simulink library "lib_fuel_converter3"  (Simulink 4.1.1)
values from neighbouring files (symbols this model uses):
  logFlag = 1    [advSACompMaskInit.m]    (also in advSACompMaskInitR13.m)
undefined symbols (not defined in the file or in its folder): air_cp, amb_tmp, cyc_mph, ex_gas_cp, fc_acc_mass, fc_base_mass, fc_c2i_th_cond, fc_c_init_tmp, fc_cl2h_eff, fc_CO2_to_FUELgps, fc_cold, fc_cold_tmp, fc_cp, fc_ct_trq, fc_emisv, fc_ext_sarea, fc_fuel_den, fc_fuel_lhv, fc_h2x_th_cond, fc_h_air_flow, fc_h_cp, fc_h_init_tmp, fc_hood_emisv, fc_hood_sarea, fc_i2x_th_cond, fc_i_init_tmp, fc_inertia, fc_map_spd, fc_map_trq, fc_max_trq, fc_nn_model_name, fc_pwr_scale, fc_spd_scale, fc_trq_scale, fc_tstat, fc_x_init_tmp, fd_ratio, gb_num_init, gb_ratio, generalName, pow, vc_idle_bool, vc_idle_spd, vc_key_on, veh_glider_mass, wh_radius
libraries: lib_fuel_converter3 x4, lib_etc x4, lib_fuel_converter x2, lib_fuel_converter2 x1
(part 1 of 9)
settings Model: LastModifiedBy=mokeefe

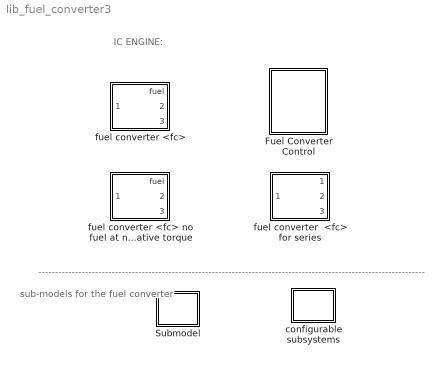
== system lib_fuel_converter3 ==
  note: --------------------------------------------------------------------------------------------------------------------
  note: sub-models
      | for the fuel converter
  note: IC ENGINE:
  Fuel Converter Control : Subsystem
      settings: RTWFcnNameOpts=Auto  RTWFileNameOpts=Auto
  Submodel : Subsystem
      settings: RTWFcnNameOpts=Auto  RTWFileNameOpts=Auto
  configurable subsystems : Subsystem
      settings: RTWFcnNameOpts=Auto  RTWFileNameOpts=Auto
  fuel converter  <fc> for series : Subsystem  mask(Stand-Alone IC ENGINE Mask (Series Hybrid)){generalName='fc', logPick=Log, initFileName={}, modCell={}, imgFileName='bdi_fc.jpg', DEBUG=OFF}
      mask prompts: generalName "General Name of this Component [char]"; logPick "Log Variables to Workspace?"; initFileName "Initialization File(s) [cell array of char]"; modCell "Modification Cell [2 column cell array of param and val]"; imgFileName "Icon image file name [char--evaluated]"
      mask init:
      | % initialization via m-file script
      | advSACompMaskInit;
      settings: RTWFcnNameOpts=Auto  RTWFileNameOpts=Auto
      mask StyleString: edit,popup(Don't Log|Log),edit,edit,edit,popup(ON|OFF)
      mask Display: image(imread(imgFileName))
  fuel converter <fc> : Subsystem  mask(Stand-Alone IC ENGINE Mask){generalName='fc', logPick=Log, initFileName={}, modCell={}, imgFileName='bdi_fc.jpg', DEBUG=OFF}
      mask prompts: generalName "General Name of this Component [char]"; logPick "Log Variables to Workspace?"; initFileName "Initialization File(s) [cell array of char]"; modCell "Modification Cell [2 column cell array of param and val]"; imgFileName "Icon image file name [char--evaluated]"
      mask init:
      | % initialization via m-file script
      | advSACompMaskInit;
      settings: RTWFcnNameOpts=Auto  RTWFileNameOpts=Auto
      mask StyleString: edit,popup(Don't Log|Log),edit,edit,edit,popup(ON|OFF)
      mask Display: image(imread(imgFileName))
  fuel converter <fc> no fuel at negative torque : Subsystem  mask(Stand-Alone IC ENGINE Mask){generalName='fc', logPick=Log, initFileName={}, modCell={}, imgFileName='bdi_fc.jpg', DEBUG=OFF}
      mask prompts: generalName "General Name of this Component [char]"; logPick "Log Variables to Workspace?"; initFileName "Initialization File(s) [cell array of char]"; modCell "Modification Cell [2 column cell array of param and val]"; imgFileName "Icon image file name [char--evaluated]"
      mask init:
      | % initialization via m-file script
      | advSACompMaskInit;
      settings: RTWFcnNameOpts=Auto  RTWFileNameOpts=Auto
      mask StyleString: edit,popup(Don't Log|Log),edit,edit,edit,popup(ON|OFF)
      mask Display: image(imread(imgFileName))

== system lib_fuel_converter3/Fuel Converter Control ==
  Fuel Converter Control conventional ic engine : Subsystem
      settings: RTWFcnNameOpts=Auto  RTWFileNameOpts=Auto

== system lib_fuel_converter3/Submodel ==
  engine inertia as a function of total vehicle inertia (generous approximation) : Subsystem  Orientation=down
      settings: RTWFcnNameOpts=Auto  RTWFileNameOpts=Auto
  veh mass calc : Subsystem
      settings: RTWFcnNameOpts=Auto  RTWFileNameOpts=Auto

== system lib_fuel_converter3/configurable subsystems ==
  fuel use and EO emis : Subsystem
      settings: RTWFcnNameOpts=Auto  RTWFileNameOpts=Auto
  fuel use and EO emis Configurable Subsystem : Subsystem  BlockChoice=fuel use and EO emis
      settings: TemplateBlock=self  MemberBlocks=fuel use and EO emis,fuel use and EO emis Neural Network Model  RTWFcnNameOpts=Auto  RTWFileNameOpts=Auto
  fuel use and EO emis Neural Network Model : Subsystem  mask{modelName=fc_nn_model_name}
      mask prompts: modelName "model no. (see help for specs)"
      mask help: Neural Network Model for Engine Fuel and Emissions Prediction
      mask init:
      | if strcmp(modelName,'1999CumminsISM370')
      |      modelNum=0;
      |      disp('Neural Net Model: 1999CumminsISM370')
      | elseif strcmp(modelName,'1994NavistarT444E')
      |      modelNum=1;
      |      disp('Neural Net Model: 1994NavistarT444E')
      | else
      |      modelNum=-1;
      |      disp('Neural Net Model: Invalid Setting!')
      |      disp('check value of fc_nn_model_name')
      | end
      settings: RTWFcnNameOpts=Auto  RTWFileNameOpts=Auto
      mask Help:
      | <h1>Neural Network Emissions Block Help</h1>
      | <h2>Introduction</h2>
      | <p>The neural network model takes engine shaft speed and torque and their time derivatives at 5 seconds and 10 seconds and predicts CO, CO2, and NOx emissions in g/s. Inputs to the model are speed (rpm) and torque (Nm). Outputs are CO, CO2, and NOx emissions in g/s.</p>
      | 
      | <p>There are neural network models trained for two engines thus far:</p>
      | <ol>
      | <li>1999 Cummins ISM 370</li>
      | <li>1994 Navistar T 444E</li>
      | </ol>
      | <p>In order to access the neural net models, one must type a string into the mask input screen. That string corresponds to:</p>
      | 
      | <table border=1>
      | <tr><td>Name</td><td>Engine</td></tr>
      | <tr><td>'1999CumminsISM370'</td><td>Cummins ISM 370</td></tr>
      | <tr><td>'1994NavistarT444E'</td><td>Navistar T 444E</td></tr>
      | </table>

== system lib_fuel_converter3/fuel converter  <fc> for series ==
  note: Internal Combustion Engine
      | for Series Powertrain
  torque and speed  req'd at engine  output shaft (Nm) : Inport  Port=1  LatchInput=off
  Model & Interface : Subsystem
      settings: RTWFcnNameOpts=Auto  RTWFileNameOpts=Auto
  fuel use : Outport  Port=1  InitialOutput=0
  EO emis info : Outport  Port=2  InitialOutput=0
  "torque and speed  avail. to driveline (Nm), (rad/s)" : Outport  Port=3  InitialOutput=0
  tag scope: fcReqOut=global, fcSensors=global
  wires:
  Model & Interface/2(fuel use) -> fuel use/1
  torque and speed  req'd at engine  output shaft (Nm)/1 -> Model & Interface/1(torque and speed  req'd at engine  output shaft (Nm))
  Model & Interface/3(EO emis info) -> EO emis info/1
  Model & Interface/4("torque and speed  avail. to driveline (Nm), (rad/s)") -> "torque and speed  avail. to driveline (Nm), (rad/s)"/1
  [fcControl] -> Model & Interface/2(control)
  Model & Interface/1(req'd out) -> [fcReqOut]
  Model & Interface/5(sensors) -> [fcSensors]

== system lib_fuel_converter3/fuel converter <fc> ==
  note: Internal Combustion Engine
  trq and spd out requested : Inport  Port=1  LatchInput=off
  Block NOTES : Subsystem
      settings: RTWFcnNameOpts=Auto  RTWFileNameOpts=Auto
      mask Display: disp('Block\nNOTES')
  IC Engine Model  &  Interface : Subsystem
      settings: RTWFcnNameOpts=Auto  RTWFileNameOpts=Auto
  help : Subsystem
      settings: OpenFcn=web(['file:\\\' which('fuel_converter.htm')]);  RTWFcnNameOpts=Auto  RTWFileNameOpts=Auto
      mask Display: image(imread('doc_man.jpg'))
  fuel : Outport  Port=1
  engine out emissions : Outport  Port=2
  trq and spd out achieved : Outport  Port=3
  tag scope: fcReqOut=global, fcSensors=global
  wires:
  trq and spd out requested/1 -> IC Engine Model  &  Interface/1(trq and spd out requested)
  [fcControl] -> IC Engine Model  &  Interface/2(control)
  IC Engine Model  &  Interface/5(sensors) -> [fcSensors]
  IC Engine Model  &  Interface/4(trq and spd out achieved) -> trq and spd out achieved/1
  IC Engine Model  &  Interface/3(engine out emissions) -> engine out emissions/1
  IC Engine Model  &  Interface/2(fuel) -> fuel/1
  IC Engine Model  &  Interface/1(req out) -> [fcReqOut]

== system lib_fuel_converter3/fuel converter <fc> no fuel at negative torque ==
  note: Internal Combustion Engine
  trq and spd out requested : Inport  Port=1  LatchInput=off
  Block NOTES : Subsystem
      settings: RTWFcnNameOpts=Auto  RTWFileNameOpts=Auto
      mask Display: disp('Block\nNOTES')
  IC Engine Model  &  Interface : Subsystem
      settings: RTWFcnNameOpts=Auto  RTWFileNameOpts=Auto
  help : Subsystem
      settings: OpenFcn=web(['file:\\\' which('fuel_converter.htm')]);  RTWFcnNameOpts=Auto  RTWFileNameOpts=Auto
      mask Display: image(imread('doc_man.jpg'))
  fuel : Outport  Port=1
  engine out emissions : Outport  Port=2
  trq and spd out achieved : Outport  Port=3
  tag scope: fcReqOut=global, fcSensors=global
  wires:
  trq and spd out requested/1 -> IC Engine Model  &  Interface/1(trq and spd out requested)
  [fcControl] -> IC Engine Model  &  Interface/2(control)
  IC Engine Model  &  Interface/5(sensors) -> [fcSensors]
  IC Engine Model  &  Interface/4(trq and spd out achieved) -> trq and spd out achieved/1
  IC Engine Model  &  Interface/3(engine out emissions) -> engine out emissions/1
  IC Engine Model  &  Interface/2(fuel) -> fuel/1
  IC Engine Model  &  Interface/1(req out) -> [fcReqOut]

== system lib_fuel_converter3/Fuel Converter Control/Fuel Converter Control conventional ic engine ==
  conventional IC engine : Subsystem
      settings: RTWFcnNameOpts=Auto  RTWFileNameOpts=Auto

== system lib_fuel_converter3/Submodel/engine inertia as a function of total vehicle inertia (generous approximation) ==
  Product : Product  Orientation=down  Inputs=*/  Multiplication=Element-wise(.*)  SaturateOnIntegerOverflow=on
  Sum : Sum  Orientation=down  Inputs=++|  SaturateOnIntegerOverflow=on
  engine inertia as a fraction of total vehicle inertia  (generous approximation)--denomenator : Fcn  Orientation=down  Expr=fc_inertia*(u*fd_ratio/wh_radius)^2
  engine inertia as a fraction of total vehicle inertia  (generous approximation)--numerator : Fcn  Orientation=down  Expr=fc_inertia*(u*fd_ratio/wh_radius)^2
  veh mass calc : lib_fuel_converter3/Submodel/veh mass calc
      settings: RTWFcnNameOpts=Auto  RTWFileNameOpts=Auto
  Out1 : Outport  Orientation=down  Port=1
  wires:
  Product/1 -> Out1/1
  Sum/1 -> Product/2
  engine inertia as a fraction of total vehicle inertia  (generous approximation)--numerator/1 -> Product/1
  engine inertia as a fraction of total vehicle inertia  (generous approximation)--denomenator/1 -> Sum/2
  veh mass calc/1 -> Sum/1
  [gear_ratio] -> engine inertia as a fraction of total vehicle inertia  (generous approximation)--denomenator/1, engine inertia as a fraction of total vehicle inertia  (generous approximation)--numerator/1

== system lib_fuel_converter3/Submodel/veh mass calc ==
  Out1 : Outport  Port=1
  wires:
  [current_veh_mass] -> Out1/1

== system lib_fuel_converter3/configurable subsystems/fuel use and EO emis ==
  T (Nm) : Inport  Port=1  LatchInput=off
  w (rad/s) : Inport  Port=2  LatchInput=off
  (gal/s) : Gain  Gain=1/fc_fuel_den*61.02/231  Multiplication=Element-wise(K.*u)  SaturateOnIntegerOverflow=on
  Block NOTES : Subsystem
      settings: RTWFcnNameOpts=Auto  RTWFileNameOpts=Auto
      mask Display: disp('Block\nNOTES')
  Demux : Demux  Outputs=2  BusSelectionMode=off
  HOT engine maps : Subsystem  TreatAsAtomicUnit=on
      settings: RTWFcnNameOpts=Auto  RTWFileNameOpts=Auto
  Integrator : Integrator  ExternalReset=none  InitialConditionSource=internal  InitialCondition=0  LimitOutput=off  UpperSaturationLimit=inf  LowerSaturationLimit=-inf  ShowSaturationPort=off  ShowStatePort=off  AbsoluteTolerance=auto
  Mux4 : Mux  Inputs=[1 4 1 1 1]
      settings: DisplayOption=none
  Mux5 : Mux  Inputs=[1 4 ]
      settings: DisplayOption=none
  Selector3 : Selector  Orientation=down  InputType=Vector  ElementSrc=Internal  Elements=2  RowSrc=Internal  Rows=1  ColumnSrc=Internal  Columns=1  InputPortWidth=4
  Terminator : Terminator
  enhancedToWorkspace1 : Subsystem  mask(enhancedToWorkspace){generalName=generalName, specificName=th_pwr, logFlag=logFlag}
      mask prompts: generalName "General Name [char-evaluated]"; specificName "Specific Name [char-literal]"; logFlag "Enable flag (1=on,0=off)"
      mask help: A wrapper for the Simulink "To Workspace" block that allows you to evaluate the name of the variable to log to workspace. This is useful to avoid the double logging errors that occur when you pull in two library models that attempt to log to the same variable.
      mask init:
      | enhancedToWsMaker
      settings: CopyFcn=breakLinkCopyFcn  RTWFcnNameOpts=Auto  RTWFileNameOpts=Auto
      mask Display: disp([generalName,'_',specificName])
  enhancedToWorkspace10 : Subsystem  mask(enhancedToWorkspace){generalName=generalName, specificName=ex_gas_tmp, logFlag=logFlag}
      mask prompts: generalName "General Name [char-evaluated]"; specificName "Specific Name [char-literal]"; logFlag "Enable flag (1=on,0=off)"
      mask help: A wrapper for the Simulink "To Workspace" block that allows you to evaluate the name of the variable to log to workspace. This is useful to avoid the double logging errors that occur when you pull in two library models that attempt to log to the same variable.
      mask init:
      | enhancedToWsMaker
      settings: CopyFcn=breakLinkCopyFcn  RTWFcnNameOpts=Auto  RTWFileNameOpts=Auto
      mask Display: disp([generalName,'_',specificName])
  enhancedToWorkspace11 : Subsystem  mask(enhancedToWorkspace){generalName=generalName, specificName=ex_th_pwr, logFlag=logFlag}
      mask prompts: generalName "General Name [char-evaluated]"; specificName "Specific Name [char-literal]"; logFlag "Enable flag (1=on,0=off)"
      mask help: A wrapper for the Simulink "To Workspace" block that allows you to evaluate the name of the variable to log to workspace. This is useful to avoid the double logging errors that occur when you pull in two library models that attempt to log to the same variable.
      mask init:
      | enhancedToWsMaker
      settings: CopyFcn=breakLinkCopyFcn  RTWFcnNameOpts=Auto  RTWFileNameOpts=Auto
      mask Display: disp([generalName,'_',specificName])
  enhancedToWorkspace12 : Subsystem  Orientation=left  mask(enhancedToWorkspace){generalName=generalName, specificName=clt_tmp, logFlag=logFlag}
      mask prompts: generalName "General Name [char-evaluated]"; specificName "Specific Name [char-literal]"; logFlag "Enable flag (1=on,0=off)"
      mask help: A wrapper for the Simulink "To Workspace" block that allows you to evaluate the name of the variable to log to workspace. This is useful to avoid the double logging errors that occur when you pull in two library models that attempt to log to the same variable.
      mask init:
      | enhancedToWsMaker
      settings: CopyFcn=breakLinkCopyFcn  RTWFcnNameOpts=Auto  RTWFileNameOpts=Auto
      mask Display: disp([generalName,'_',specificName])
  enhancedToWorkspace2 : Subsystem  mask(enhancedToWorkspace){generalName=generalName, specificName=o2_flow, logFlag=logFlag}
      mask prompts: generalName "General Name [char-evaluated]"; specificName "Specific Name [char-literal]"; logFlag "Enable flag (1=on,0=off)"
      mask help: A wrapper for the Simulink "To Workspace" block that allows you to evaluate the name of the variable to log to workspace. This is useful to avoid the double logging errors that occur when you pull in two library models that attempt to log to the same variable.
      mask init:
      | enhancedToWsMaker
      settings: CopyFcn=breakLinkCopyFcn  RTWFcnNameOpts=Auto  RTWFileNameOpts=Auto
      mask Display: disp([generalName,'_',specificName])
  enhancedToWorkspace3 : Subsystem  mask(enhancedToWorkspace){generalName=generalName, specificName=r_th_pwr, logFlag=logFlag}
      mask prompts: generalName "General Name [char-evaluated]"; specificName "Specific Name [char-literal]"; logFlag "Enable flag (1=on,0=off)"
      mask help: A wrapper for the Simulink "To Workspace" block that allows you to evaluate the name of the variable to log to workspace. This is useful to avoid the double logging errors that occur when you pull in two library models that attempt to log to the same variable.
      mask init:
      | enhancedToWsMaker
      settings: CopyFcn=breakLinkCopyFcn  RTWFcnNameOpts=Auto  RTWFileNameOpts=Auto
      mask Display: disp([generalName,'_',specificName])
  enhancedToWorkspace5 : Subsystem  mask(enhancedToWorkspace){generalName=generalName, specificName=h_th_pwr, logFlag=logFlag}
      mask prompts: generalName "General Name [char-evaluated]"; specificName "Specific Name [char-literal]"; logFlag "Enable flag (1=on,0=off)"
      mask help: A wrapper for the Simulink "To Workspace" block that allows you to evaluate the name of the variable to log to workspace. This is useful to avoid the double logging errors that occur when you pull in two library models that attempt to log to the same variable.
      mask init:
      | enhancedToWsMaker
      settings: CopyFcn=breakLinkCopyFcn  RTWFcnNameOpts=Auto  RTWFileNameOpts=Auto
      mask Display: disp([generalName,'_',specificName])
  enhancedToWorkspace6 : Subsystem  mask(enhancedToWorkspace){generalName=generalName, specificName=tmp, logFlag=logFlag}
      mask prompts: generalName "General Name [char-evaluated]"; specificName "Specific Name [char-literal]"; logFlag "Enable flag (1=on,0=off)"
      mask help: A wrapper for the Simulink "To Workspace" block that allows you to evaluate the name of the variable to log to workspace. This is useful to avoid the double logging errors that occur when you pull in two library models that attempt to log to the same variable.
      mask init:
      | enhancedToWsMaker
      settings: CopyFcn=breakLinkCopyFcn  RTWFcnNameOpts=Auto  RTWFileNameOpts=Auto
      mask Display: disp([generalName,'_',specificName])
  enhancedToWorkspace7 : Subsystem  mask(enhancedToWorkspace){generalName=generalName, specificName=fuel_rate, logFlag=logFlag}
      mask prompts: generalName "General Name [char-evaluated]"; specificName "Specific Name [char-literal]"; logFlag "Enable flag (1=on,0=off)"
      mask help: A wrapper for the Simulink "To Workspace" block that allows you to evaluate the name of the variable to log to workspace. This is useful to avoid the double logging errors that occur when you pull in two library models that attempt to log to the same variable.
      mask init:
      | enhancedToWsMaker
      settings: CopyFcn=breakLinkCopyFcn  RTWFcnNameOpts=Auto  RTWFileNameOpts=Auto
      mask Display: disp([generalName,'_',specificName])
  enhancedToWorkspace8 : Subsystem  mask(enhancedToWorkspace){generalName=generalName, specificName=emis_eo, logFlag=logFlag}
      mask prompts: generalName "General Name [char-evaluated]"; specificName "Specific Name [char-literal]"; logFlag "Enable flag (1=on,0=off)"
      mask help: A wrapper for the Simulink "To Workspace" block that allows you to evaluate the name of the variable to log to workspace. This is useful to avoid the double logging errors that occur when you pull in two library models that attempt to log to the same variable.
      mask init:
      | enhancedToWsMaker
      settings: CopyFcn=breakLinkCopyFcn  RTWFcnNameOpts=Auto  RTWFileNameOpts=Auto
      mask Display: disp([generalName,'_',specificName])
  enhancedToWorkspace9 : Subsystem  mask(enhancedToWorkspace){generalName=generalName, specificName=ex_gas_flow, logFlag=logFlag}
      mask prompts: generalName "General Name [char-evaluated]"; specificName "Specific Name [char-literal]"; logFlag "Enable flag (1=on,0=off)"
      mask help: A wrapper for the Simulink "To Workspace" block that allows you to evaluate the name of the variable to log to workspace. This is useful to avoid the double logging errors that occur when you pull in two library models that attempt to log to the same variable.
      mask init:
      | enhancedToWsMaker
      settings: CopyFcn=breakLinkCopyFcn  RTWFcnNameOpts=Auto  RTWFileNameOpts=Auto
      mask Display: disp([generalName,'_',specificName])
  fc temp : Subsystem
      settings: RTWFcnNameOpts=Auto  RTWFileNameOpts=Auto
  fc temp correct : Subsystem  TreatAsAtomicUnit=on
      settings: RTWFcnNameOpts=Auto  RTWFileNameOpts=Auto
  cumulative fuel  use (gal) : Outport  Port=1  InitialOutput=0
  "FC ON?, EOem, MFex, Tex, O2ex" : Outport  Port=2  InitialOutput=0
  Vv,Tfc : Outport  Port=3  InitialOutput=0
  tag scope: fc_clt_tmp=scoped
  wires:
  [key_on] -> fc temp/2(key ON?)
  [engine_on] -> fc temp/3(fc ON?), fc temp correct/Enable, Mux4/1, HOT engine maps/Enable
  fc temp correct/2(EO emis (g/s)) -> Mux4/2, enhancedToWorkspace8/1(In1)
  Demux/2 -> enhancedToWorkspace5/1(In1)
  Demux/1 -> enhancedToWorkspace3/1(In1)
  fc temp/2(Qfc r,h) -> Demux/1
  HOT engine maps/1(fc heat (W)) -> fc temp/4(Qfc (W)), enhancedToWorkspace1/1(In1)
  Selector3/1 -> fc temp correct/1(Coolant T (C)), [fc_clt_tmp], enhancedToWorkspace12/1(In1)
  HOT engine maps/7(ex heat (W)) -> enhancedToWorkspace11/1(In1)
  fc temp/1(Tfc_old  (C)) -> Terminator/1
  fc temp/3(Tfc  (C)) -> Mux5/2, enhancedToWorkspace6/1(In1), Selector3/1
  HOT engine maps/3(HOT emis (g/s)) -> fc temp correct/3(HOT emis (g/s))
  HOT engine maps/2(HOT fuel use (g/s)) -> fc temp correct/2(HOT fuel use (g/s))
  (gal/s)/1 -> Integrator/1
  Integrator/1 -> cumulative fuel  use (gal)/1
  HOT engine maps/5(Ex Gas Temp (C)) -> Mux4/4, enhancedToWorkspace10/1(In1)
  HOT engine maps/4(Ex Gas Flow (g/s)) -> Mux4/3, enhancedToWorkspace9/1(In1)
  [v_prev] -> fc temp/1(veh spd (m/s)), Mux5/1
  Mux5/1 -> Vv,Tfc/1
  Mux4/1 -> "FC ON?, EOem, MFex, Tex, O2ex"/1
  w (rad/s)/1 -> fc temp correct/5(w (rad/s)), HOT engine maps/2(w (rad/s))
  T (Nm)/1 -> fc temp correct/4(T (Nm)), HOT engine maps/1(T (Nm))
  HOT engine maps/6(O2 exhaust (g/s)) -> Mux4/5, enhancedToWorkspace2/1(In1)
  fc temp correct/1(fuel use (g/s)) -> (gal/s)/1, enhancedToWorkspace7/1(In1)

== system lib_fuel_converter3/configurable subsystems/fuel use and EO emis Configurable Subsystem ==
  T (Nm) : Inport  Port=1  LatchInput=off
  w (rad/s) : Inport  Port=2  LatchInput=off
  fuel use and EO emis : lib_fuel_converter3/configurable subsystems/fuel use and EO emis
      settings: RTWFcnNameOpts=Auto  RTWFileNameOpts=Auto
  cumulative fuel  use (gal) : Outport  Port=1
  "FC ON?, EOem, MFex, Tex, O2ex" : Outport  Port=2
  Vv,Tfc : Outport  Port=3
  wires:
  T (Nm)/1 -> fuel use and EO emis/1
  w (rad/s)/1 -> fuel use and EO emis/2
  fuel use and EO emis/1 -> cumulative fuel  use (gal)/1
  fuel use and EO emis/2 -> "FC ON?, EOem, MFex, Tex, O2ex"/1
  fuel use and EO emis/3 -> Vv,Tfc/1

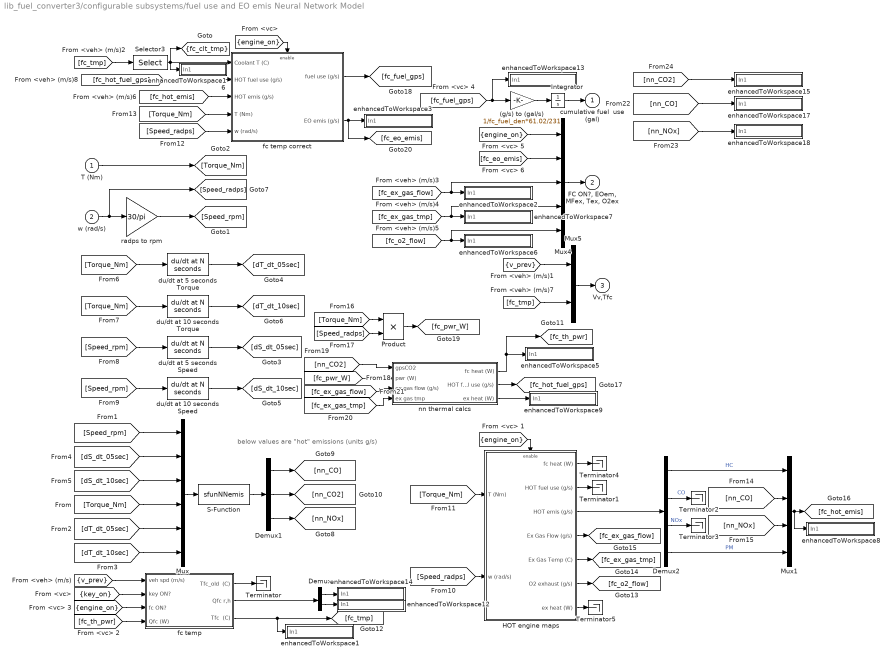
== system lib_fuel_converter3/configurable subsystems/fuel use and EO emis Neural Network Model ==
  note: below values are "hot" emissions
      | (units g/s)
  T (Nm) : Inport  Port=1  LatchInput=off
  w (rad/s) : Inport  Port=2  LatchInput=off
  (g/s) to (gal/s) : Gain  Gain=1/fc_fuel_den*61.02/231  Multiplication=Element-wise(K.*u)  SaturateOnIntegerOverflow=on
  Demux : Demux  Outputs=2  BusSelectionMode=off
  Demux1 : Demux  Outputs=3  BusSelectionMode=off
  Demux2 : Demux  Outputs=4  BusSelectionMode=off
  HOT engine maps : Subsystem  TreatAsAtomicUnit=on
      settings: RTWFcnNameOpts=Auto  RTWFileNameOpts=Auto
  Integrator : Integrator  ExternalReset=none  InitialConditionSource=internal  InitialCondition=0  LimitOutput=off  UpperSaturationLimit=inf  LowerSaturationLimit=-inf  ShowSaturationPort=off  ShowStatePort=off  AbsoluteTolerance=auto
  Mux : Mux  Inputs=6
  Mux1 : Mux  Inputs=4
  Mux4 : Mux  Inputs=[1 4 1 1 1]
      settings: DisplayOption=none
  Mux5 : Mux  Inputs=[1 4 ]
      settings: DisplayOption=none
  Product : Product  Inputs=2  Multiplication=Element-wise(.*)  SaturateOnIntegerOverflow=on
  S-Function : S-Function  FunctionName=sfunNNemis  Parameters=modelNum  PortCounts=[]  SFunctionModules=''
  Selector3 : Selector  InputType=Vector  ElementSrc=Internal  Elements=2  RowSrc=Internal  Rows=1  ColumnSrc=Internal  Columns=1  InputPortWidth=4
  Terminator{,1..5} (6 alike) : Terminator
  du/dt at 10 seconds Speed : lib_etc/du//dt at N seconds  delay=10
  du/dt at 10 seconds Torque : lib_etc/du//dt at N seconds  delay=10
  du/dt at 5 seconds Speed : lib_etc/du//dt at N seconds  delay=5
  du/dt at 5 seconds Torque : lib_etc/du//dt at N seconds  delay=5
  enhancedToWorkspace1 : Subsystem  mask(enhancedToWorkspace){generalName=generalName, specificName=tmp, logFlag=logFlag}
      mask prompts: generalName "General Name [char-evaluated]"; specificName "Specific Name [char-literal]"; logFlag "Enable flag (1=on,0=off)"
      mask help: A wrapper for the Simulink "To Workspace" block that allows you to evaluate the name of the variable to log to workspace. This is useful to avoid the double logging errors that occur when you pull in two library models that attempt to log to the same variable.
      mask init:
      | enhancedToWsMaker
      settings: CopyFcn=breakLinkCopyFcn  RTWFcnNameOpts=Auto  RTWFileNameOpts=Auto
      mask Display: disp([generalName,'_',specificName])
  enhancedToWorkspace12 : Subsystem  mask(enhancedToWorkspace){generalName=generalName, specificName=h_th_pwr, logFlag=logFlag}
      mask prompts: generalName "General Name [char-evaluated]"; specificName "Specific Name [char-literal]"; logFlag "Enable flag (1=on,0=off)"
      mask help: A wrapper for the Simulink "To Workspace" block that allows you to evaluate the name of the variable to log to workspace. This is useful to avoid the double logging errors that occur when you pull in two library models that attempt to log to the same variable.
      mask init:
      | enhancedToWsMaker
      settings: CopyFcn=breakLinkCopyFcn  RTWFcnNameOpts=Auto  RTWFileNameOpts=Auto
      mask Display: disp([generalName,'_',specificName])
  enhancedToWorkspace13 : Subsystem  mask(enhancedToWorkspace){generalName=generalName, specificName=fuel_rate, logFlag=logFlag}
      mask prompts: generalName "General Name [char-evaluated]"; specificName "Specific Name [char-literal]"; logFlag "Enable flag (1=on,0=off)"
      mask help: A wrapper for the Simulink "To Workspace" block that allows you to evaluate the name of the variable to log to workspace. This is useful to avoid the double logging errors that occur when you pull in two library models that attempt to log to the same variable.
      mask init:
      | enhancedToWsMaker
      settings: CopyFcn=breakLinkCopyFcn  RTWFcnNameOpts=Auto  RTWFileNameOpts=Auto
      mask Display: disp([generalName,'_',specificName])
  enhancedToWorkspace14 : Subsystem  mask(enhancedToWorkspace){generalName=generalName, specificName=r_th_pwr, logFlag=logFlag}
      mask prompts: generalName "General Name [char-evaluated]"; specificName "Specific Name [char-literal]"; logFlag "Enable flag (1=on,0=off)"
      mask help: A wrapper for the Simulink "To Workspace" block that allows you to evaluate the name of the variable to log to workspace. This is useful to avoid the double logging errors that occur when you pull in two library models that attempt to log to the same variable.
      mask init:
      | enhancedToWsMaker
      settings: CopyFcn=breakLinkCopyFcn  RTWFcnNameOpts=Auto  RTWFileNameOpts=Auto
      mask Display: disp([generalName,'_',specificName])
  enhancedToWorkspace15 : Subsystem  mask(enhancedToWorkspace){generalName=generalName, specificName=nn_CO2, logFlag=logFlag}
      mask prompts: generalName "General Name [char-evaluated]"; specificName "Specific Name [char-literal]"; logFlag "Enable flag (1=on,0=off)"
      mask help: A wrapper for the Simulink "To Workspace" block that allows you to evaluate the name of the variable to log to workspace. This is useful to avoid the double logging errors that occur when you pull in two library models that attempt to log to the same variable.
      mask init:
      | enhancedToWsMaker
      settings: CopyFcn=breakLinkCopyFcn  RTWFcnNameOpts=Auto  RTWFileNameOpts=Auto
      mask Display: disp([generalName,'_',specificName])
  enhancedToWorkspace16 : Subsystem  mask(enhancedToWorkspace){generalName=generalName, specificName=clt_tmp, logFlag=logFlag}
      mask prompts: generalName "General Name [char-evaluated]"; specificName "Specific Name [char-literal]"; logFlag "Enable flag (1=on,0=off)"
      mask help: A wrapper for the Simulink "To Workspace" block that allows you to evaluate the name of the variable to log to workspace. This is useful to avoid the double logging errors that occur when you pull in two library models that attempt to log to the same variable.
      mask init:
      | enhancedToWsMaker
      settings: CopyFcn=breakLinkCopyFcn  RTWFcnNameOpts=Auto  RTWFileNameOpts=Auto
      mask Display: disp([generalName,'_',specificName])
  enhancedToWorkspace17 : Subsystem  mask(enhancedToWorkspace){generalName=generalName, specificName=nn_CO, logFlag=logFlag}
      mask prompts: generalName "General Name [char-evaluated]"; specificName "Specific Name [char-literal]"; logFlag "Enable flag (1=on,0=off)"
      mask help: A wrapper for the Simulink "To Workspace" block that allows you to evaluate the name of the variable to log to workspace. This is useful to avoid the double logging errors that occur when you pull in two library models that attempt to log to the same variable.
      mask init:
      | enhancedToWsMaker
      settings: CopyFcn=breakLinkCopyFcn  RTWFcnNameOpts=Auto  RTWFileNameOpts=Auto
      mask Display: disp([generalName,'_',specificName])
  enhancedToWorkspace18 : Subsystem  mask(enhancedToWorkspace){generalName=generalName, specificName=nn_NOx, logFlag=logFlag}
      mask prompts: generalName "General Name [char-evaluated]"; specificName "Specific Name [char-literal]"; logFlag "Enable flag (1=on,0=off)"
      mask help: A wrapper for the Simulink "To Workspace" block that allows you to evaluate the name of the variable to log to workspace. This is useful to avoid the double logging errors that occur when you pull in two library models that attempt to log to the same variable.
      mask init:
      | enhancedToWsMaker
      settings: CopyFcn=breakLinkCopyFcn  RTWFcnNameOpts=Auto  RTWFileNameOpts=Auto
      mask Display: disp([generalName,'_',specificName])
  enhancedToWorkspace2 : Subsystem  mask(enhancedToWorkspace){generalName=generalName, specificName=ex_gas_flow, logFlag=logFlag}
      mask prompts: generalName "General Name [char-evaluated]"; specificName "Specific Name [char-literal]"; logFlag "Enable flag (1=on,0=off)"
      mask help: A wrapper for the Simulink "To Workspace" block that allows you to evaluate the name of the variable to log to workspace. This is useful to avoid the double logging errors that occur when you pull in two library models that attempt to log to the same variable.
      mask init:
      | enhancedToWsMaker
      settings: CopyFcn=breakLinkCopyFcn  RTWFcnNameOpts=Auto  RTWFileNameOpts=Auto
      mask Display: disp([generalName,'_',specificName])
  enhancedToWorkspace3 : Subsystem  mask(enhancedToWorkspace){generalName=generalName, specificName=emis_eo, logFlag=logFlag}
      mask prompts: generalName "General Name [char-evaluated]"; specificName "Specific Name [char-literal]"; logFlag "Enable flag (1=on,0=off)"
      mask help: A wrapper for the Simulink "To Workspace" block that allows you to evaluate the name of the variable to log to workspace. This is useful to avoid the double logging errors that occur when you pull in two library models that attempt to log to the same variable.
      mask init:
      | enhancedToWsMaker
      settings: CopyFcn=breakLinkCopyFcn  RTWFcnNameOpts=Auto  RTWFileNameOpts=Auto
      mask Display: disp([generalName,'_',specificName])
  enhancedToWorkspace5 : Subsystem  mask(enhancedToWorkspace){generalName=generalName, specificName=th_pwr, logFlag=logFlag}
      mask prompts: generalName "General Name [char-evaluated]"; specificName "Specific Name [char-literal]"; logFlag "Enable flag (1=on,0=off)"
      mask help: A wrapper for the Simulink "To Workspace" block that allows you to evaluate the name of the variable to log to workspace. This is useful to avoid the double logging errors that occur when you pull in two library models that attempt to log to the same variable.
      mask init:
      | enhancedToWsMaker
      settings: CopyFcn=breakLinkCopyFcn  RTWFcnNameOpts=Auto  RTWFileNameOpts=Auto
      mask Display: disp([generalName,'_',specificName])
  enhancedToWorkspace6 : Subsystem  mask(enhancedToWorkspace){generalName=generalName, specificName=o2_flow, logFlag=logFlag}
      mask prompts: generalName "General Name [char-evaluated]"; specificName "Specific Name [char-literal]"; logFlag "Enable flag (1=on,0=off)"
      mask help: A wrapper for the Simulink "To Workspace" block that allows you to evaluate the name of the variable to log to workspace. This is useful to avoid the double logging errors that occur when you pull in two library models that attempt to log to the same variable.
      mask init:
      | enhancedToWsMaker
      settings: CopyFcn=breakLinkCopyFcn  RTWFcnNameOpts=Auto  RTWFileNameOpts=Auto
      mask Display: disp([generalName,'_',specificName])
  enhancedToWorkspace7 : Subsystem  mask(enhancedToWorkspace){generalName=generalName, specificName=ex_gas_tmp, logFlag=logFlag}
      mask prompts: generalName "General Name [char-evaluated]"; specificName "Specific Name [char-literal]"; logFlag "Enable flag (1=on,0=off)"
      mask help: A wrapper for the Simulink "To Workspace" block that allows you to evaluate the name of the variable to log to workspace. This is useful to avoid the double logging errors that occur when you pull in two library models that attempt to log to the same variable.
      mask init:
      | enhancedToWsMaker
      settings: CopyFcn=breakLinkCopyFcn  RTWFcnNameOpts=Auto  RTWFileNameOpts=Auto
      mask Display: disp([generalName,'_',specificName])
  enhancedToWorkspace8 : Subsystem  mask(enhancedToWorkspace){generalName=generalName, specificName=hotemis_eo, logFlag=logFlag}
      mask prompts: generalName "General Name [char-evaluated]"; specificName "Specific Name [char-literal]"; logFlag "Enable flag (1=on,0=off)"
      mask help: A wrapper for the Simulink "To Workspace" block that allows you to evaluate the name of the variable to log to workspace. This is useful to avoid the double logging errors that occur when you pull in two library models that attempt to log to the same variable.
      mask init:
      | enhancedToWsMaker
      settings: CopyFcn=breakLinkCopyFcn  RTWFcnNameOpts=Auto  RTWFileNameOpts=Auto
      mask Display: disp([generalName,'_',specificName])
  enhancedToWorkspace9 : Subsystem  mask(enhancedToWorkspace){generalName=generalName, specificName=ex_th_pwr, logFlag=logFlag}
      mask prompts: generalName "General Name [char-evaluated]"; specificName "Specific Name [char-literal]"; logFlag "Enable flag (1=on,0=off)"
      mask help: A wrapper for the Simulink "To Workspace" block that allows you to evaluate the name of the variable to log to workspace. This is useful to avoid the double logging errors that occur when you pull in two library models that attempt to log to the same variable.
      mask init:
      | enhancedToWsMaker
      settings: CopyFcn=breakLinkCopyFcn  RTWFcnNameOpts=Auto  RTWFileNameOpts=Auto
      mask Display: disp([generalName,'_',specificName])
  fc temp : Subsystem
      settings: RTWFcnNameOpts=Auto  RTWFileNameOpts=Auto
  fc temp correct : Subsystem  TreatAsAtomicUnit=on
      settings: RTWFcnNameOpts=Auto  RTWFileNameOpts=Auto
  nn thermal calcs : Subsystem
      settings: RTWFcnNameOpts=Auto  RTWFileNameOpts=Auto
  radps to rpm : Gain  Gain=30/pi  Multiplication=Element-wise(K.*u)  SaturateOnIntegerOverflow=on
  cumulative fuel  use (gal) : Outport  Port=1  InitialOutput=0
  "FC ON?, EOem, MFex, Tex, O2ex" : Outport  Port=2  InitialOutput=0
  Vv,Tfc : Outport  Port=3  InitialOutput=0
  tag scope: fc_clt_tmp=scoped
  wires:
  [engine_on] -> fc temp correct/Enable
  fc temp correct/2(EO emis (g/s)) -> [fc_eo_emis], enhancedToWorkspace3/1(In1)
  Selector3/1 -> fc temp correct/1(Coolant T (C)), [fc_clt_tmp], enhancedToWorkspace16/1(In1)
  Mux5/1 -> Vv,Tfc/1
  w (rad/s)/1 -> radps to rpm/1, [Speed_radps]
  radps to rpm/1 -> [Speed_rpm]
  T (Nm)/1 -> [Torque_Nm]
  [Torque_Nm] -> du/dt at 5 seconds Torque/1
  [Torque_Nm] -> du/dt at 10 seconds Torque/1
  [Speed_rpm] -> du/dt at 5 seconds Speed/1
  [Speed_rpm] -> du/dt at 10 seconds Speed/1
  du/dt at 5 seconds Torque/1 -> [dT_dt_05sec]
  du/dt at 5 seconds Speed/1 -> [dS_dt_05sec]
  du/dt at 10 seconds Speed/1 -> [dS_dt_10sec]
  du/dt at 10 seconds Torque/1 -> [dT_dt_10sec]
  Mux/1 -> S-Function/1
  S-Function/1 -> Demux1/1
  Demux1/1 -> [nn_CO]
  Demux1/2 -> [nn_CO2]
  Demux1/3 -> [nn_NOx]
  [v_prev] -> Mux5/1
  [fc_tmp] -> Selector3/1
  [key_on] -> fc temp/2(key ON?)
  Demux/2 -> enhancedToWorkspace12/1(In1)
  Demux/1 -> enhancedToWorkspace14/1(In1)
  fc temp/2(Qfc r,h) -> Demux/1
  fc temp/1(Tfc_old  (C)) -> Terminator/1
  fc temp/3(Tfc  (C)) -> [fc_tmp], enhancedToWorkspace1/1(In1)
  [v_prev] -> fc temp/1(veh spd (m/s))
  [fc_th_pwr] -> fc temp/4(Qfc (W))
  [engine_on] -> fc temp/3(fc ON?)
  [fc_hot_emis] -> fc temp correct/3(HOT emis (g/s))
  HOT engine maps/5(Ex Gas Temp (C)) -> [fc_ex_gas_tmp]
  HOT engine maps/4(Ex Gas Flow (g/s)) -> [fc_ex_gas_flow]
  HOT engine maps/6(O2 exhaust (g/s)) -> [fc_o2_flow]
  [Torque_Nm] -> HOT engine maps/1(T (Nm))
  [Speed_radps] -> HOT engine maps/2(w (rad/s))
  [engine_on] -> HOT engine maps/Enable
  HOT engine maps/2(HOT fuel use (g/s)) -> Terminator1/1
  [fc_tmp] -> Mux5/2
  [fc_ex_gas_flow] -> Mux4/3, enhancedToWorkspace2/1(In1)
  [fc_ex_gas_tmp] -> Mux4/4, enhancedToWorkspace7/1(In1)
  [fc_o2_flow] -> Mux4/5, enhancedToWorkspace6/1(In1)
  Mux4/1 -> "FC ON?, EOem, MFex, Tex, O2ex"/1
  [Speed_rpm] -> Mux/1
  [dS_dt_05sec] -> Mux/2
  [dS_dt_10sec] -> Mux/3
  [Torque_Nm] -> Mux/4
  [dT_dt_05sec] -> Mux/5
  [dT_dt_10sec] -> Mux/6
  [Torque_Nm] -> fc temp correct/4(T (Nm))
  [Speed_radps] -> fc temp correct/5(w (rad/s))
  Mux1/1 -> [fc_hot_emis], enhancedToWorkspace8/1(In1)
  HOT engine maps/3(HOT emis (g/s)) -> Demux2/1
  Demux2/1 -> Mux1/1  "HC"
  Demux2/4 -> Mux1/4  "PM"
  Demux2/2 -> Terminator2/1  "CO"
  Demux2/3 -> Terminator3/1  "NOx"
  [nn_CO] -> Mux1/2
  [nn_NOx] -> Mux1/3
  HOT engine maps/1(fc heat (W)) -> Terminator4/1
  HOT engine maps/7(ex heat (W)) -> Terminator5/1
  nn thermal calcs/3(ex heat (W)) -> enhancedToWorkspace9/1(In1)
  nn thermal calcs/1(fc heat (W)) -> [fc_th_pwr], enhancedToWorkspace5/1(In1)
  nn thermal calcs/2(HOT fuel use (g/s)) -> [fc_hot_fuel_gps]
  [fc_hot_fuel_gps] -> fc temp correct/2(HOT fuel use (g/s))
  fc temp correct/1(fuel use (g/s)) -> [fc_fuel_gps]
  (g/s) to (gal/s)/1 -> Integrator/1
  Integrator/1 -> cumulative fuel  use (gal)/1
  [fc_fuel_gps] -> (g/s) to (gal/s)/1, enhancedToWorkspace13/1(In1)
  [Torque_Nm] -> Product/1
  [Speed_radps] -> Product/2
  Product/1 -> [fc_pwr_W]
  [nn_CO2] -> nn thermal calcs/1(gpsCO2)
  [fc_pwr_W] -> nn thermal calcs/2(pwr (W))
  [fc_ex_gas_flow] -> nn thermal calcs/3(ex gas flow (g/s))
  [fc_ex_gas_tmp] -> nn thermal calcs/4(ex gas tmp)
  [engine_on] -> Mux4/1
  [fc_eo_emis] -> Mux4/2
  [nn_CO2] -> enhancedToWorkspace15/1(In1)
  [nn_CO] -> enhancedToWorkspace17/1(In1)
  [nn_NOx] -> enhancedToWorkspace18/1(In1)

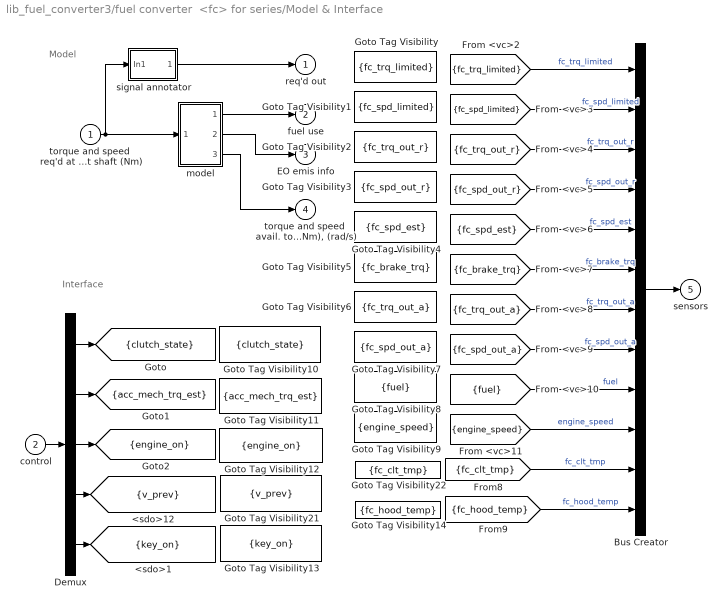
== system lib_fuel_converter3/fuel converter  <fc> for series/Model & Interface ==
  note: Model
  note: Interface
  torque and speed  req'd at engine  output shaft (Nm) : Inport  Port=1  LatchInput=off
  control : Inport  Port=2  LatchInput=off
  Bus Creator : BusCreator  Inputs=12
  Demux : Demux  Outputs=5  BusSelectionMode=off
  Goto Tag Visibility : GotoTagVisibility  GotoTag=fc_trq_limited
  Goto Tag Visibility1 : GotoTagVisibility  GotoTag=fc_spd_limited
  Goto Tag Visibility10 : GotoTagVisibility  GotoTag=clutch_state
  Goto Tag Visibility11 : GotoTagVisibility  GotoTag=acc_mech_trq_est
  Goto Tag Visibility12 : GotoTagVisibility  GotoTag=engine_on
  Goto Tag Visibility13 : GotoTagVisibility  GotoTag=key_on
  Goto Tag Visibility14 : GotoTagVisibility  GotoTag=fc_hood_temp
  Goto Tag Visibility2 : GotoTagVisibility  GotoTag=fc_trq_out_r
  Goto Tag Visibility21 : GotoTagVisibility  GotoTag=v_prev
  Goto Tag Visibility22 : GotoTagVisibility  GotoTag=fc_clt_tmp
  Goto Tag Visibility3 : GotoTagVisibility  GotoTag=fc_spd_out_r
  Goto Tag Visibility4 : GotoTagVisibility  GotoTag=fc_spd_est
  Goto Tag Visibility5 : GotoTagVisibility  GotoTag=fc_brake_trq
  Goto Tag Visibility6 : GotoTagVisibility  GotoTag=fc_trq_out_a
  Goto Tag Visibility7 : GotoTagVisibility  GotoTag=fc_spd_out_a
  Goto Tag Visibility8 : GotoTagVisibility  GotoTag=fuel
  Goto Tag Visibility9 : GotoTagVisibility  GotoTag=engine_speed
  model : Subsystem
      settings: RTWFcnNameOpts=Auto  RTWFileNameOpts=Auto
  signal annotator : Subsystem
      settings: RTWFcnNameOpts=Auto  RTWFileNameOpts=Auto
  req'd out : Outport  Port=1  InitialOutput=0
  fuel use : Outport  Port=2  InitialOutput=0
  EO emis info : Outport  Port=3  InitialOutput=0
  "torque and speed  avail. to driveline (Nm), (rad/s)" : Outport  Port=4  InitialOutput=0
  sensors : Outport  Port=5  InitialOutput=0
  tag scope: acc_mech_trq_est=scoped, clutch_state=scoped, engine_on=scoped, key_on=scoped, v_prev=scoped
  wires:
  model/1(fuel use) -> fuel use/1
  torque and speed  req'd at engine  output shaft (Nm)/1 -> model/1(torque and speed  req'd at engine  output shaft (Nm)), signal annotator/1(In1)
  model/2(EO emis info) -> EO emis info/1
  model/3("torque and speed  avail. to driveline (Nm), (rad/s)") -> "torque and speed  avail. to driveline (Nm), (rad/s)"/1
  signal annotator/1(Out1) -> req'd out/1
  Bus Creator/1 -> sensors/1
  Demux/1 -> [clutch_state]
  Demux/2 -> [acc_mech_trq_est]
  Demux/3 -> [engine_on]
  control/1 -> Demux/1
  [fc_trq_limited] -> Bus Creator/1  "fc_trq_limited"
  [fc_spd_limited] -> Bus Creator/2  "fc_spd_limited"
  [fc_trq_out_r] -> Bus Creator/3  "fc_trq_out_r"
  [fc_spd_out_r] -> Bus Creator/4  "fc_spd_out_r"
  [fc_spd_est] -> Bus Creator/5  "fc_spd_est"
  [fc_brake_trq] -> Bus Creator/6  "fc_brake_trq"
  [fc_trq_out_a] -> Bus Creator/7  "fc_trq_out_a"
  [fc_spd_out_a] -> Bus Creator/8  "fc_spd_out_a"
  [fuel] -> Bus Creator/9  "fuel"
  [engine_speed] -> Bus Creator/10  "engine_speed"
  [fc_hood_temp] -> Bus Creator/12  "fc_hood_temp"
  [fc_clt_tmp] -> Bus Creator/11  "fc_clt_tmp"
  Demux/4 -> [v_prev]
  Demux/5 -> [key_on]

== system lib_fuel_converter3/fuel converter <fc>/Block NOTES ==
  note: This block models the internal combustion engine, and includes inertia effects,
      | performance limits, accessory loads, and temperature transient effects on fuel
      | use, engine-out emissions, and catalyst efficiency.  There are 'leads' to the
      | engine controller here, which controller determines whether the engine is on.

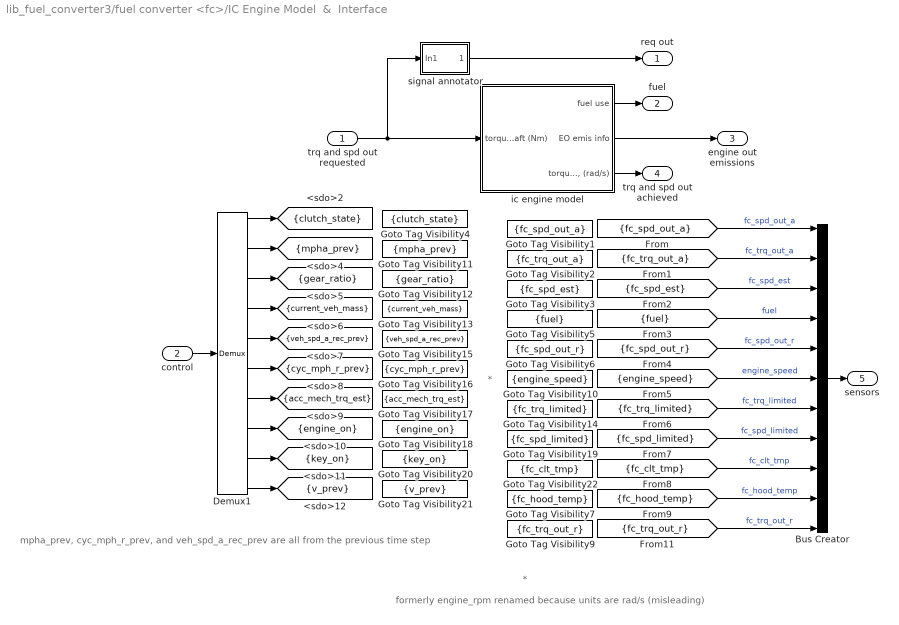
== system lib_fuel_converter3/fuel converter <fc>/IC Engine Model  &  Interface ==
  note: mpha_prev, cyc_mph_r_prev, and veh_spd_a_rec_prev
      | are all from the previous time step
  note: *
  note: *
  note: formerly
      | engine_rpm
      | renamed because
      | units are rad/s
      |  (misleading)
  trq and spd out requested : Inport  Port=1  LatchInput=off
  control : Inport  Port=2  LatchInput=off
  Bus Creator : BusCreator  Inputs=11
  Demux1 : Demux  Outputs=10  BusSelectionMode=off
  Goto Tag Visibility1 : GotoTagVisibility  GotoTag=fc_spd_out_a
  Goto Tag Visibility10 : GotoTagVisibility  GotoTag=engine_speed
  Goto Tag Visibility11 : GotoTagVisibility  GotoTag=mpha_prev
  Goto Tag Visibility12 : GotoTagVisibility  GotoTag=gear_ratio
  Goto Tag Visibility13 : GotoTagVisibility  GotoTag=current_veh_mass
  Goto Tag Visibility14 : GotoTagVisibility  GotoTag=fc_trq_limited
  Goto Tag Visibility15 : GotoTagVisibility  GotoTag=veh_spd_a_rec_prev
  Goto Tag Visibility16 : GotoTagVisibility  GotoTag=cyc_mph_r_prev
  Goto Tag Visibility17 : GotoTagVisibility  GotoTag=acc_mech_trq_est
  Goto Tag Visibility18 : GotoTagVisibility  GotoTag=engine_on
  Goto Tag Visibility19 : GotoTagVisibility  GotoTag=fc_spd_limited
  Goto Tag Visibility2 : GotoTagVisibility  GotoTag=fc_trq_out_a
  Goto Tag Visibility20 : GotoTagVisibility  GotoTag=key_on
  Goto Tag Visibility21 : GotoTagVisibility  GotoTag=v_prev
  Goto Tag Visibility22 : GotoTagVisibility  GotoTag=fc_clt_tmp
  Goto Tag Visibility3 : GotoTagVisibility  GotoTag=fc_spd_est
  Goto Tag Visibility4 : GotoTagVisibility  GotoTag=clutch_state
  Goto Tag Visibility5 : GotoTagVisibility  GotoTag=fuel
  Goto Tag Visibility6 : GotoTagVisibility  GotoTag=fc_spd_out_r
  Goto Tag Visibility7 : GotoTagVisibility  GotoTag=fc_hood_temp
  Goto Tag Visibility9 : GotoTagVisibility  GotoTag=fc_trq_out_r
  ic engine model : Subsystem
      settings: RTWFcnNameOpts=Auto  RTWFileNameOpts=Auto
  signal annotator : Subsystem
      settings: RTWFcnNameOpts=Auto  RTWFileNameOpts=Auto
  req out : Outport  Port=1
  fuel : Outport  Port=2
  engine out emissions : Outport  Port=3
  trq and spd out achieved : Outport  Port=4
  sensors : Outport  Port=5
  tag scope: acc_mech_trq_est=scoped, clutch_state=scoped, current_veh_mass=scoped, cyc_mph_r_prev=scoped, engine_on=scoped, gear_ratio=scoped, key_on=scoped, mpha_prev=scoped, v_prev=scoped, veh_spd_a_rec_prev=scoped
  wires:
  [fc_trq_out_r] -> Bus Creator/11  "fc_trq_out_r"
  [fc_hood_temp] -> Bus Creator/10  "fc_hood_temp"
  [fc_clt_tmp] -> Bus Creator/9  "fc_clt_tmp"
  [fc_spd_limited] -> Bus Creator/8  "fc_spd_limited"
  [fc_trq_limited] -> Bus Creator/7  "fc_trq_limited"
  [engine_speed] -> Bus Creator/6  "engine_speed"
  [fc_spd_out_r] -> Bus Creator/5  "fc_spd_out_r"
  [fuel] -> Bus Creator/4  "fuel"
  [fc_spd_est] -> Bus Creator/3  "fc_spd_est"
  [fc_trq_out_a] -> Bus Creator/2  "fc_trq_out_a"
  [fc_spd_out_a] -> Bus Creator/1  "fc_spd_out_a"
  Demux1/1 -> [clutch_state]
  Demux1/2 -> [mpha_prev]
  Demux1/3 -> [gear_ratio]
  Demux1/4 -> [current_veh_mass]
  Demux1/5 -> [veh_spd_a_rec_prev]
  Demux1/6 -> [cyc_mph_r_prev]
  Demux1/7 -> [acc_mech_trq_est]
  Demux1/8 -> [engine_on]
  Demux1/9 -> [key_on]
  Demux1/10 -> [v_prev]
  trq and spd out requested/1 -> ic engine model/1(torque and speed  req'd at engine  output shaft (Nm)), signal annotator/1(In1)
  ic engine model/1(fuel use) -> fuel/1
  ic engine model/2(EO emis info) -> engine out emissions/1
  ic engine model/3("torque and speed  avail. to driveline (Nm), (rad/s)") -> trq and spd out achieved/1
  control/1 -> Demux1/1
  Bus Creator/1 -> sensors/1
  signal annotator/1(Out1) -> req out/1

== system lib_fuel_converter3/fuel converter <fc>/help ==

== system lib_fuel_converter3/fuel converter <fc> no fuel at negative torque/Block NOTES ==
  note: This block models the internal combustion engine, and includes inertia effects,
      | performance limits, accessory loads, and temperature transient effects on fuel
      | use, engine-out emissions, and catalyst efficiency.  There are 'leads' to the
      | engine controller here, which controller determines whether the engine is on.
